simulink model "mconversionFixPointSupport2"  (Simulink 6.0)
settings: Solver=FixedStepDiscrete  StartTime=0.0  StopTime=10.0  RelTol=1e-3
PreLoadFcn:
  | hconversionFixPointSupport2
undefined symbols (not defined in the file or in its folder): dden, tsamp
libraries: simulink x10
settings Model: Creator=myunt  LastModifiedBy=myunt  ExtModeAutoUpdateStatusClock=off
settings DebuggingCC: CheckExecutionContextPreStartOutputMsg=on  CheckExecutionContextRuntimeOutputMsg=on

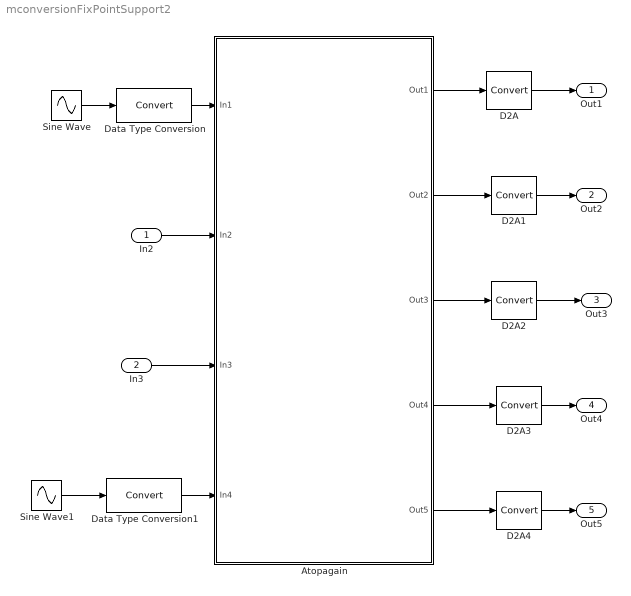
== system mconversionFixPointSupport2 ==
  In2 : Inport  LatchInput=off
  In3 : Inport  Port=2  LatchInput=off
  Atopagain : Subsystem  TreatAsAtomicUnit=on  PropExecContextAcrossSSBoundary=on
  D2A{,1..4} (5 alike) : DataTypeConversion  OutDataTypeMode=double
  Data Type Conversion : DataTypeConversion
  Data Type Conversion1 : DataTypeConversion
  Sine Wave : Sin  SineType=Sample based  SampleTime=tsamp
  Sine Wave1 : Sin  SineType=Sample based  SampleTime=tsamp
  Out1 : Outport
  Out2 : Outport  Port=2
  Out3 : Outport  Port=3
  Out4 : Outport  Port=4
  Out5 : Outport  Port=5
  wires:
  Sine Wave/1 -> Data Type Conversion/1
  Atopagain/1(Out1) -> D2A/1
  D2A/1 -> Out1/1
  Atopagain/2(Out2) -> D2A1/1
  D2A1/1 -> Out2/1
  In3/1 -> Atopagain/3(In3)
  D2A2/1 -> Out3/1
  Atopagain/4(Out4) -> D2A3/1
  D2A3/1 -> Out4/1
  In2/1 -> Atopagain/2(In2)
  Data Type Conversion1/1 -> Atopagain/4(In4)
  Atopagain/3(Out3) -> D2A2/1
  Atopagain/5(Out5) -> D2A4/1
  D2A4/1 -> Out5/1
  Data Type Conversion/1 -> Atopagain/1(In1)
  Sine Wave1/1 -> Data Type Conversion1/1

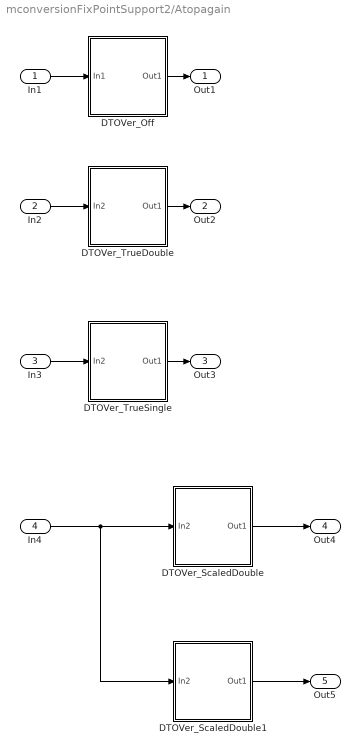
== system mconversionFixPointSupport2/Atopagain ==
  In1 : Inport  LatchInput=off
  In2 : Inport  Port=2  LatchInput=off
  In3 : Inport  Port=3  LatchInput=off
  In4 : Inport  Port=4  LatchInput=off
  DTOVer_Off : Subsystem  PropExecContextAcrossSSBoundary=on
  DTOVer_ScaledDouble : Subsystem  PropExecContextAcrossSSBoundary=on  DataTypeOverride=ScaledDoubles
  DTOVer_ScaledDouble1 : Subsystem  PropExecContextAcrossSSBoundary=on  DataTypeOverride=ScaledDoubles
  DTOVer_TrueDouble : Subsystem  PropExecContextAcrossSSBoundary=on  DataTypeOverride=TrueDoubles
  DTOVer_TrueSingle : Subsystem  PropExecContextAcrossSSBoundary=on  DataTypeOverride=TrueSingles
  Out1 : Outport
  Out2 : Outport  Port=2
  Out3 : Outport  Port=3
  Out4 : Outport  Port=4
  Out5 : Outport  Port=5
  wires:
  In1/1 -> DTOVer_Off/1(In1)
  DTOVer_Off/1(Out1) -> Out1/1
  In2/1 -> DTOVer_TrueDouble/1(In2)
  DTOVer_TrueDouble/1(Out1) -> Out2/1
  In3/1 -> DTOVer_TrueSingle/1(In2)
  DTOVer_TrueSingle/1(Out1) -> Out3/1
  In4/1 -> DTOVer_ScaledDouble/1(In2), DTOVer_ScaledDouble1/1(In2)
  DTOVer_ScaledDouble/1(Out1) -> Out4/1
  DTOVer_ScaledDouble1/1(Out1) -> Out5/1

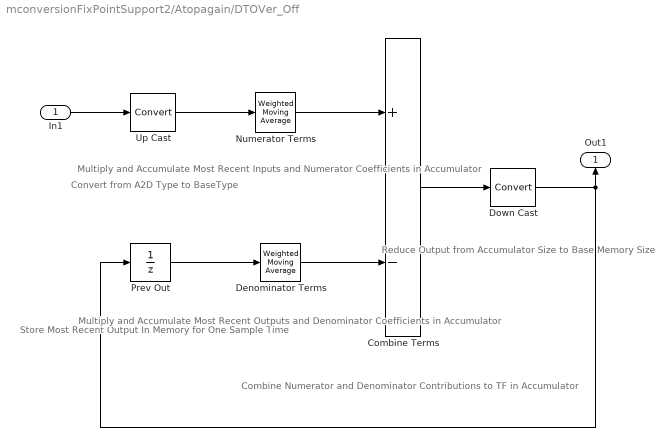
== system mconversionFixPointSupport2/Atopagain/DTOVer_Off ==
  note: Reduce Output from
      | Accumulator Size to
      | Base Memory Size
  note: Combine Numerator
      | and Denominator
      | Contributions to TF
      | in Accumulator
  note: Store Most
      | Recent Output
      | In Memory for
      | One Sample Time
  note: Multiply and Accumulate
      | Most Recent Outputs and
      | Denominator Coefficients
      | in Accumulator
  note: Multiply and Accumulate
      | Most Recent Inputs and
      | Numerator Coefficients
      | in Accumulator
  note: Convert from
      | A2D Type
      | to BaseType
  In1 : Inport  DataType=Specify via dialog  OutScaling=2^-8  LatchInput=off
  Combine Terms : Sum  Inputs=+-  OutDataTypeMode=Specify via dialog  OutDataType=AccumType  OutScaling=2^(-12)  SaturateOnIntegerOverflow=on
  Denominator Terms : simulink/Discrete/Weighted Moving Average  mgainval=dden(2:length(dden))  vinit=0.0  samptime=tsamp  GainDataTypeScalingMode=Specify via dialog  GainDataType=BaseType  MatRadixGroup=Best Precision: Element-wise  GainScaling=2^-14  OutputDataTypeScalingMode=Specify via dialog  OutDataType=AccumType  OutScaling=2^(-12)  DoSatur=on
  Down Cast : DataTypeConversion  OutDataTypeMode=Specify via dialog  OutDataType=BaseType  OutScaling=2^(-5)  SaturateOnIntegerOverflow=on
  Numerator Terms : simulink/Discrete/Weighted Moving Average  mgainval=dnum  vinit=0.0  samptime=tsamp  GainDataTypeScalingMode=Specify via dialog  GainDataType=BaseType  MatRadixGroup=Best Precision: Element-wise  GainScaling=2^-14  OutputDataTypeScalingMode=Specify via dialog  OutDataType=AccumType  OutScaling=2^(-12)  DoSatur=on
  Prev Out : UnitDelay  X0=0.0  SampleTime=tsamp
  Up Cast : DataTypeConversion  OutDataTypeMode=Specify via dialog  OutDataType=BaseType  OutScaling=2^(-14)  SaturateOnIntegerOverflow=on
  Out1 : Outport  Orientation=up  InitialOutput=0
  wires:
  Down Cast/1 -> Out1/1, Prev Out/1
  In1/1 -> Up Cast/1
  Up Cast/1 -> Numerator Terms/1
  Prev Out/1 -> Denominator Terms/1
  Numerator Terms/1 -> Combine Terms/1
  Denominator Terms/1 -> Combine Terms/2
  Combine Terms/1 -> Down Cast/1

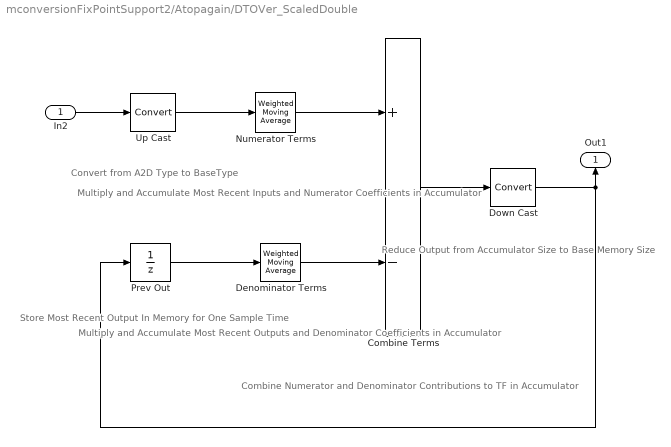
== system mconversionFixPointSupport2/Atopagain/DTOVer_ScaledDouble ==
  note: Convert from
      | A2D Type
      | to BaseType
  note: Multiply and Accumulate
      | Most Recent Inputs and
      | Numerator Coefficients
      | in Accumulator
  note: Multiply and Accumulate
      | Most Recent Outputs and
      | Denominator Coefficients
      | in Accumulator
  note: Store Most
      | Recent Output
      | In Memory for
      | One Sample Time
  note: Combine Numerator
      | and Denominator
      | Contributions to TF
      | in Accumulator
  note: Reduce Output from
      | Accumulator Size to
      | Base Memory Size
  In2 : Inport  DataType=Specify via dialog  OutScaling=2^-8  LatchInput=off
  Combine Terms : Sum  Inputs=+-  OutDataTypeMode=Specify via dialog  OutDataType=AccumType  OutScaling=2^(-12)  SaturateOnIntegerOverflow=on
  Denominator Terms : simulink/Discrete/Weighted Moving Average  mgainval=dden(2:length(dden))  vinit=0.0  samptime=tsamp  GainDataTypeScalingMode=Specify via dialog  GainDataType=BaseType  MatRadixGroup=Best Precision: Element-wise  GainScaling=2^-14  OutputDataTypeScalingMode=Specify via dialog  OutDataType=AccumType  OutScaling=2^(-12)  DoSatur=on
  Down Cast : DataTypeConversion  OutDataTypeMode=Specify via dialog  OutDataType=BaseType  OutScaling=2^(-5)  SaturateOnIntegerOverflow=on
  Numerator Terms : simulink/Discrete/Weighted Moving Average  mgainval=dnum  vinit=0.0  samptime=tsamp  GainDataTypeScalingMode=Specify via dialog  GainDataType=BaseType  MatRadixGroup=Best Precision: Element-wise  GainScaling=2^-14  OutputDataTypeScalingMode=Specify via dialog  OutDataType=AccumType  OutScaling=2^(-12)  DoSatur=on
  Prev Out : UnitDelay  X0=0.0  SampleTime=tsamp
  Up Cast : DataTypeConversion  OutDataTypeMode=Specify via dialog  OutDataType=BaseType  OutScaling=2^(-14)  SaturateOnIntegerOverflow=on
  Out1 : Outport  Orientation=up  InitialOutput=0
  wires:
  Combine Terms/1 -> Down Cast/1
  Denominator Terms/1 -> Combine Terms/2
  Numerator Terms/1 -> Combine Terms/1
  Prev Out/1 -> Denominator Terms/1
  Up Cast/1 -> Numerator Terms/1
  In2/1 -> Up Cast/1
  Down Cast/1 -> Prev Out/1, Out1/1

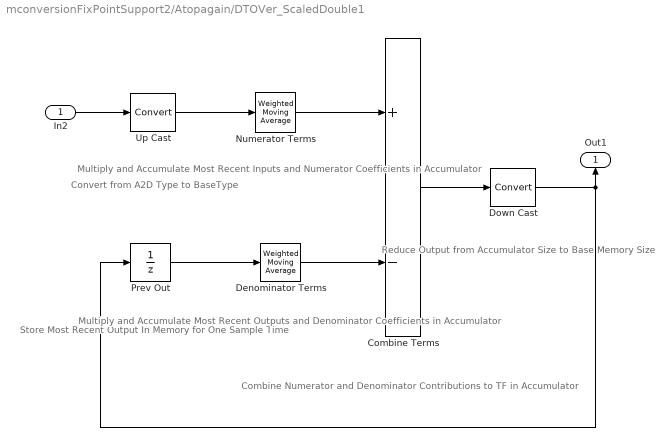
== system mconversionFixPointSupport2/Atopagain/DTOVer_ScaledDouble1 ==
  note: Reduce Output from
      | Accumulator Size to
      | Base Memory Size
  note: Combine Numerator
      | and Denominator
      | Contributions to TF
      | in Accumulator
  note: Store Most
      | Recent Output
      | In Memory for
      | One Sample Time
  note: Multiply and Accumulate
      | Most Recent Outputs and
      | Denominator Coefficients
      | in Accumulator
  note: Multiply and Accumulate
      | Most Recent Inputs and
      | Numerator Coefficients
      | in Accumulator
  note: Convert from
      | A2D Type
      | to BaseType
  In2 : Inport  DataType=Specify via dialog  OutScaling=2^-8  LatchInput=off
  Combine Terms : Sum  Inputs=+-  OutDataTypeMode=Specify via dialog  OutDataType=AccumType  OutScaling=2^(-12)  SaturateOnIntegerOverflow=on
  Denominator Terms : simulink/Discrete/Weighted Moving Average  mgainval=dden(2:length(dden))  vinit=0.0  samptime=tsamp  GainDataTypeScalingMode=Specify via dialog  GainDataType=BaseType  MatRadixGroup=Best Precision: Element-wise  GainScaling=2^-14  OutputDataTypeScalingMode=Specify via dialog  OutDataType=AccumType  OutScaling=2^(-12)  DoSatur=on
  Down Cast : DataTypeConversion  OutDataTypeMode=Specify via dialog  OutDataType=BaseType  OutScaling=2^(-5)  SaturateOnIntegerOverflow=on
  Numerator Terms : simulink/Discrete/Weighted Moving Average  mgainval=dnum  vinit=0.0  samptime=tsamp  GainDataTypeScalingMode=Specify via dialog  GainDataType=BaseType  MatRadixGroup=Best Precision: Element-wise  GainScaling=2^-14  OutputDataTypeScalingMode=Specify via dialog  OutDataType=AccumType  OutScaling=2^(-12)  DoSatur=on
  Prev Out : UnitDelay  X0=0.0  SampleTime=tsamp
  Up Cast : DataTypeConversion  OutDataTypeMode=Specify via dialog  OutDataType=BaseType  OutScaling=2^(-14)  SaturateOnIntegerOverflow=on
  Out1 : Outport  Orientation=up  InitialOutput=0
  wires:
  Down Cast/1 -> Out1/1, Prev Out/1
  In2/1 -> Up Cast/1
  Up Cast/1 -> Numerator Terms/1
  Prev Out/1 -> Denominator Terms/1
  Numerator Terms/1 -> Combine Terms/1
  Denominator Terms/1 -> Combine Terms/2
  Combine Terms/1 -> Down Cast/1

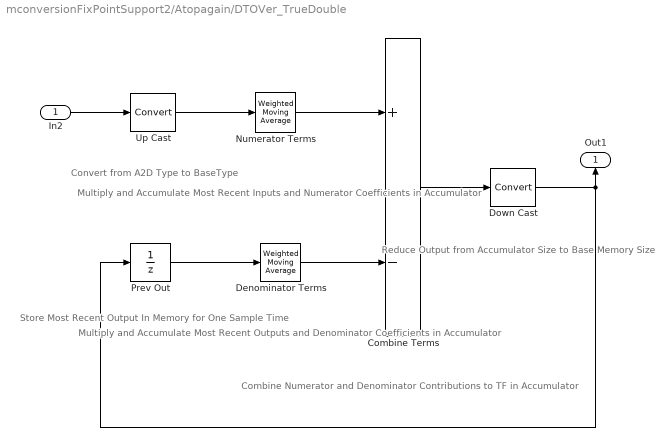
== system mconversionFixPointSupport2/Atopagain/DTOVer_TrueDouble ==
  note: Convert from
      | A2D Type
      | to BaseType
  note: Multiply and Accumulate
      | Most Recent Inputs and
      | Numerator Coefficients
      | in Accumulator
  note: Multiply and Accumulate
      | Most Recent Outputs and
      | Denominator Coefficients
      | in Accumulator
  note: Store Most
      | Recent Output
      | In Memory for
      | One Sample Time
  note: Combine Numerator
      | and Denominator
      | Contributions to TF
      | in Accumulator
  note: Reduce Output from
      | Accumulator Size to
      | Base Memory Size
  In2 : Inport  DataType=Specify via dialog  OutScaling=2^-8  LatchInput=off
  Combine Terms : Sum  Inputs=+-  OutDataTypeMode=Specify via dialog  OutDataType=AccumType  OutScaling=2^(-12)  SaturateOnIntegerOverflow=on
  Denominator Terms : simulink/Discrete/Weighted Moving Average  mgainval=dden(2:length(dden))  vinit=0.0  samptime=tsamp  GainDataTypeScalingMode=Specify via dialog  GainDataType=BaseType  MatRadixGroup=Best Precision: Element-wise  GainScaling=2^-14  OutputDataTypeScalingMode=Specify via dialog  OutDataType=AccumType  OutScaling=2^(-12)  DoSatur=on
  Down Cast : DataTypeConversion  OutDataTypeMode=Specify via dialog  OutDataType=BaseType  OutScaling=2^(-5)  SaturateOnIntegerOverflow=on
  Numerator Terms : simulink/Discrete/Weighted Moving Average  mgainval=dnum  vinit=0.0  samptime=tsamp  GainDataTypeScalingMode=Specify via dialog  GainDataType=BaseType  MatRadixGroup=Best Precision: Element-wise  GainScaling=2^-14  OutputDataTypeScalingMode=Specify via dialog  OutDataType=AccumType  OutScaling=2^(-12)  DoSatur=on
  Prev Out : UnitDelay  X0=0.0  SampleTime=tsamp
  Up Cast : DataTypeConversion  OutDataTypeMode=Specify via dialog  OutDataType=BaseType  OutScaling=2^(-14)  SaturateOnIntegerOverflow=on
  Out1 : Outport  Orientation=up  InitialOutput=0
  wires:
  Combine Terms/1 -> Down Cast/1
  Denominator Terms/1 -> Combine Terms/2
  Numerator Terms/1 -> Combine Terms/1
  Prev Out/1 -> Denominator Terms/1
  Up Cast/1 -> Numerator Terms/1
  In2/1 -> Up Cast/1
  Down Cast/1 -> Prev Out/1, Out1/1

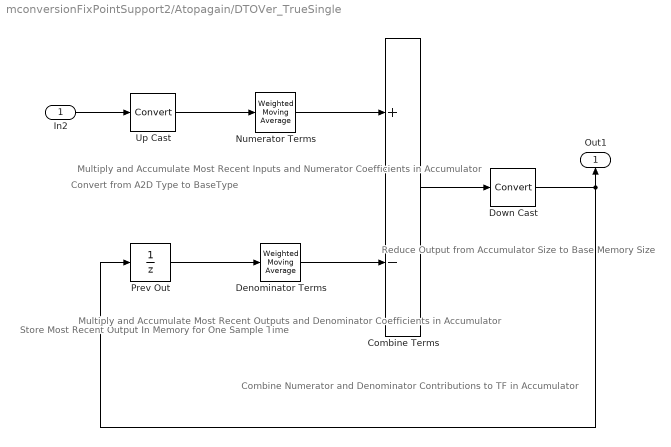
== system mconversionFixPointSupport2/Atopagain/DTOVer_TrueSingle ==
  note: Reduce Output from
      | Accumulator Size to
      | Base Memory Size
  note: Combine Numerator
      | and Denominator
      | Contributions to TF
      | in Accumulator
  note: Store Most
      | Recent Output
      | In Memory for
      | One Sample Time
  note: Multiply and Accumulate
      | Most Recent Outputs and
      | Denominator Coefficients
      | in Accumulator
  note: Multiply and Accumulate
      | Most Recent Inputs and
      | Numerator Coefficients
      | in Accumulator
  note: Convert from
      | A2D Type
      | to BaseType
  In2 : Inport  DataType=Specify via dialog  OutScaling=2^-8  LatchInput=off
  Combine Terms : Sum  Inputs=+-  OutDataTypeMode=Specify via dialog  OutDataType=AccumType  OutScaling=2^(-12)  SaturateOnIntegerOverflow=on
  Denominator Terms : simulink/Discrete/Weighted Moving Average  mgainval=dden(2:length(dden))  vinit=0.0  samptime=tsamp  GainDataTypeScalingMode=Specify via dialog  GainDataType=BaseType  MatRadixGroup=Best Precision: Element-wise  GainScaling=2^-14  OutputDataTypeScalingMode=Specify via dialog  OutDataType=AccumType  OutScaling=2^(-12)  DoSatur=on
  Down Cast : DataTypeConversion  OutDataTypeMode=Specify via dialog  OutDataType=BaseType  OutScaling=2^(-5)  SaturateOnIntegerOverflow=on
  Numerator Terms : simulink/Discrete/Weighted Moving Average  mgainval=dnum  vinit=0.0  samptime=tsamp  GainDataTypeScalingMode=Specify via dialog  GainDataType=BaseType  MatRadixGroup=Best Precision: Element-wise  GainScaling=2^-14  OutputDataTypeScalingMode=Specify via dialog  OutDataType=AccumType  OutScaling=2^(-12)  DoSatur=on
  Prev Out : UnitDelay  X0=0.0  SampleTime=tsamp
  Up Cast : DataTypeConversion  OutDataTypeMode=Specify via dialog  OutDataType=BaseType  OutScaling=2^(-14)  SaturateOnIntegerOverflow=on
  Out1 : Outport  Orientation=up  InitialOutput=0
  wires:
  Down Cast/1 -> Out1/1, Prev Out/1
  In2/1 -> Up Cast/1
  Up Cast/1 -> Numerator Terms/1
  Prev Out/1 -> Denominator Terms/1
  Numerator Terms/1 -> Combine Terms/1
  Denominator Terms/1 -> Combine Terms/2
  Combine Terms/1 -> Down Cast/1
